simulink model "BMSController"  (R2026b)
undefined symbols (not defined in the file): BalNotActWait, BalOffWait, BalOnWait, BatteryLUT, contactorTime, currentFactor, CV_Gain, DiscIntNeverNeededParam, flgEnBalancing, HighTempLimit, I_cc, LowTempLimit, MaxCellVoltThrsld, MaxChrgCurrLim, MaxDchrgCurrLim, noCurrent, OverCellVoltageLimit, PlntBattChrgMax, PlntBattNumCellPar, PlntBattNumCellSer, PlntBattSocInit, PlntBattTempInitDegC, SnsrFltThld, TargetDeltaV, timeoutContactor, timeoutCurrent, UnderCellVoltageLimit, voltThreshold, vRatio
settings Model: Creator=The MathWorks, Inc.  LastModifiedBy=The MathWorks, Inc.

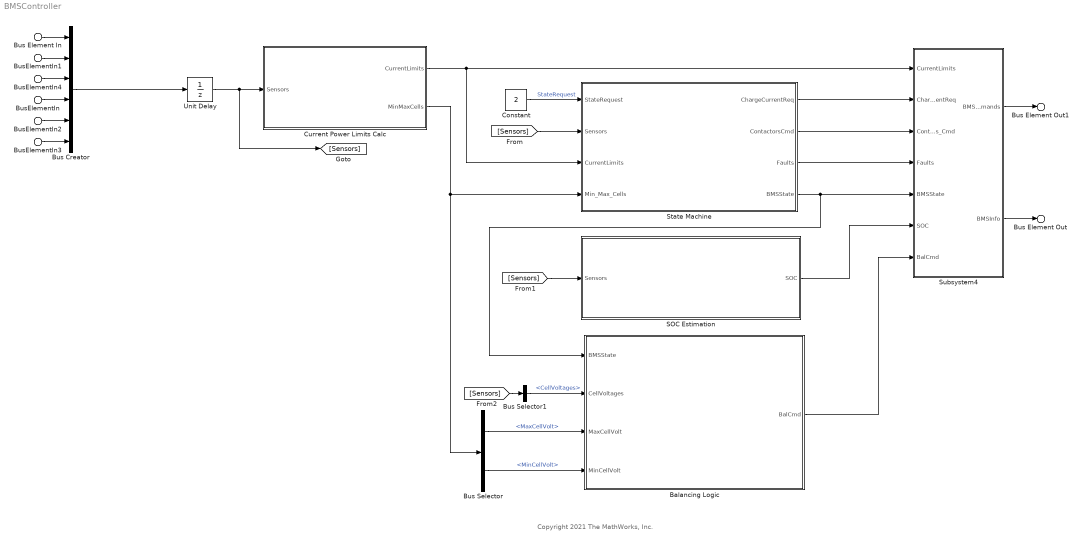
== system BMSController ==
  note: Copyright 2021 The MathWorks, Inc.
  Bus Element In : Inport  PortName=BMSSensors  Element=CellVoltages
  BusElementIn : Inport  PortName=BMSSensors  Element=CellTemperatures
  BusElementIn1 : Inport  PortName=BMSSensors  Element=PackVoltage
  BusElementIn2 : Inport  PortName=BMSSensors  Element=VoutChgr
  BusElementIn3 : Inport  PortName=BMSSensors  Element=VoutInvtr
  BusElementIn4 : Inport  PortName=BMSSensors  Element=PackCurrent
  Balancing Logic : Subsystem
  Bus Creator : BusCreator  Inputs=6
  Bus Selector : BusSelector  OutputSignals=MaxCellVolt,MinCellVolt
  Bus Selector1 : BusSelector  OutputSignals=CellVoltages
  Constant : Constant  Value=2  OutDataTypeStr=single  SampleTime=-1
  Current Power Limits Calc : Subsystem
  SOC Estimation : Subsystem
  State Machine : Subsystem
  Subsystem4 : Subsystem
  Unit Delay : UnitDelay  InitialCondition=struct('CellVoltages',3.6*ones(1, PlntBattNumCellSer),'PackVoltage',3.6*PlntBattNumCellSer,'PackCurrent',0,'CellTemperatures',PlntBattTempInitDegC*ones(1,PlntBattNumCellSer),'VoutChgr',0,'VoutInvtr',0)  SampleTime=-1
  Bus Element Out : Outport  PortName=BMSInfo
  Bus Element Out1 : Outport  Port=2  PortName=BMSCmd
  wires:
  State Machine/4(BMSState) -> Balancing Logic/1(BMSState), Subsystem4/5(BMSState)
  Constant/1 -> State Machine/1(StateRequest)  "StateRequest"
  Bus Selector1/1 -> Balancing Logic/2(CellVoltages)  "<CellVoltages>"
  SOC Estimation/1(SOC) -> Subsystem4/6(SOC)
  Balancing Logic/1(BalCmd) -> Subsystem4/7(BalCmd)
  Subsystem4/1(BMSCommands) -> Bus Element Out1/1
  Subsystem4/2(BMSInfo) -> Bus Element Out/1
  Current Power Limits Calc/1(CurrentLimits) -> State Machine/3(CurrentLimits), Subsystem4/1(CurrentLimits)
  State Machine/2(ContactorsCmd) -> Subsystem4/3(Contactors_Cmd)
  State Machine/1(ChargeCurrentReq) -> Subsystem4/2(ChargeCurrentReq)
  State Machine/3(Faults) -> Subsystem4/4(Faults)
  [Sensors] -> State Machine/2(Sensors)
  Current Power Limits Calc/2(MinMaxCells) -> State Machine/4(Min_Max_Cells), Bus Selector/1
  Bus Selector/1 -> Balancing Logic/3(MaxCellVolt)  "<MaxCellVolt>"
  Bus Selector/2 -> Balancing Logic/4(MinCellVolt)  "<MinCellVolt>"
  [Sensors] -> Bus Selector1/1
  Unit Delay/1 -> Current Power Limits Calc/1(Sensors), [Sensors]
  BusElementIn2/1 -> Bus Creator/5
  BusElementIn/1 -> Bus Creator/4
  Bus Element In/1 -> Bus Creator/1
  BusElementIn1/1 -> Bus Creator/2
  BusElementIn3/1 -> Bus Creator/6
  BusElementIn4/1 -> Bus Creator/3
  Bus Creator/1 -> Unit Delay/1
  [Sensors] -> SOC Estimation/1(Sensors)

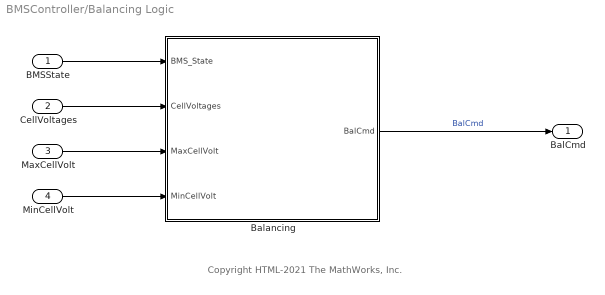
== system BMSController/Balancing Logic ==
  note: Copyright HTML-2021 The MathWorks, Inc.
  BMSState : Inport  OutDataTypeStr=single  PortDimensions=1  SampleTime=[5,0]
  CellVoltages : Inport  Port=2  OutDataTypeStr=single  PortDimensions=PlntBattNumCellSer  SampleTime=[5,0]
  MaxCellVolt : Inport  Port=3  OutDataTypeStr=single
  MinCellVolt : Inport  Port=4  OutDataTypeStr=single
  Balancing : Stateflow chart  TreatAsAtomicUnit=on  VariantControl=(default)
  BalCmd : Outport  OutDataTypeStr=boolean  PortDimensions=[1, PlntBattNumCellSer]  SampleTime=[5,0]  VectorParamsAs1DForOutWhenUnconnected=off
  wires:
  MinCellVolt/1 -> Balancing/4(MinCellVolt)
  MaxCellVolt/1 -> Balancing/3(MaxCellVolt)
  Balancing/1(BalCmd) -> BalCmd/1  "BalCmd"
  BMSState/1 -> Balancing/1(BMS_State)
  CellVoltages/1 -> Balancing/2(CellVoltages)

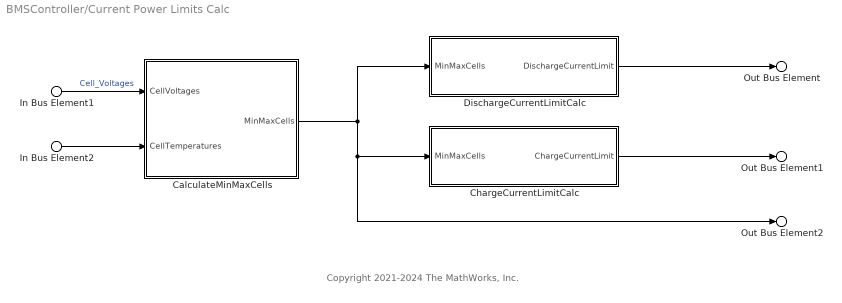
== system BMSController/Current Power Limits Calc ==
  note: Copyright 2021-2024 The MathWorks, Inc.
  In Bus Element1 : Inport  PortName=Sensors  Element=CellVoltages
  In Bus Element2 : Inport  PortName=Sensors  Element=CellTemperatures
  CalculateMinMaxCells : Subsystem
  ChargeCurrentLimitCalc : Subsystem
  DischargeCurrentLimitCalc : Subsystem
  Out Bus Element : Outport  PortName=CurrentLimits  Element=DischargeCurrentLimit
  Out Bus Element1 : Outport  PortName=CurrentLimits  Element=ChargeCurrentLimit
  Out Bus Element2 : Outport  Port=2  PortName=MinMaxCells
  wires:
  In Bus Element1/1 -> CalculateMinMaxCells/1(CellVoltages)  "Cell_Voltages"
  ChargeCurrentLimitCalc/1(ChargeCurrentLimit) -> Out Bus Element1/1
  In Bus Element2/1 -> CalculateMinMaxCells/2(CellTemperatures)
  CalculateMinMaxCells/1(MinMaxCells) -> Out Bus Element2/1, ChargeCurrentLimitCalc/1(MinMaxCells), DischargeCurrentLimitCalc/1(MinMaxCells)
  DischargeCurrentLimitCalc/1(DischargeCurrentLimit) -> Out Bus Element/1

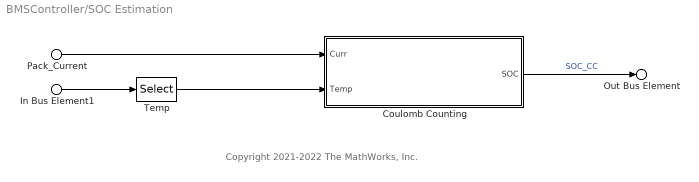
== system BMSController/SOC Estimation ==
  note: Copyright 2021-2022 The MathWorks, Inc.
  Pack_Current : Inport  PortName=Sensors  Element=PackCurrent
  In Bus Element1 : Inport  PortName=Sensors  Element=CellTemperatures
  Coulomb Counting : Subsystem  Variant=on  VariantControlMode=label  VariantControl=SocAlgo==1  LabelModeActiveChoice=Constant Capacity
  Temp : Selector  InputPortWidth=PlntBattNumCellSer  IndexOptions=Index vector (dialog)  Indices=1  OutputSizes=1  RuntimeRangeChecks=off
  Out Bus Element : Outport  PortName=SOC  Element=SOC_CC
  wires:
  Temp/1 -> Coulomb Counting/2(Temp)
  Pack_Current/1 -> Coulomb Counting/1(Curr)
  In Bus Element1/1 -> Temp/1
  Coulomb Counting/1(SOC) -> Out Bus Element/1  "SOC_CC"

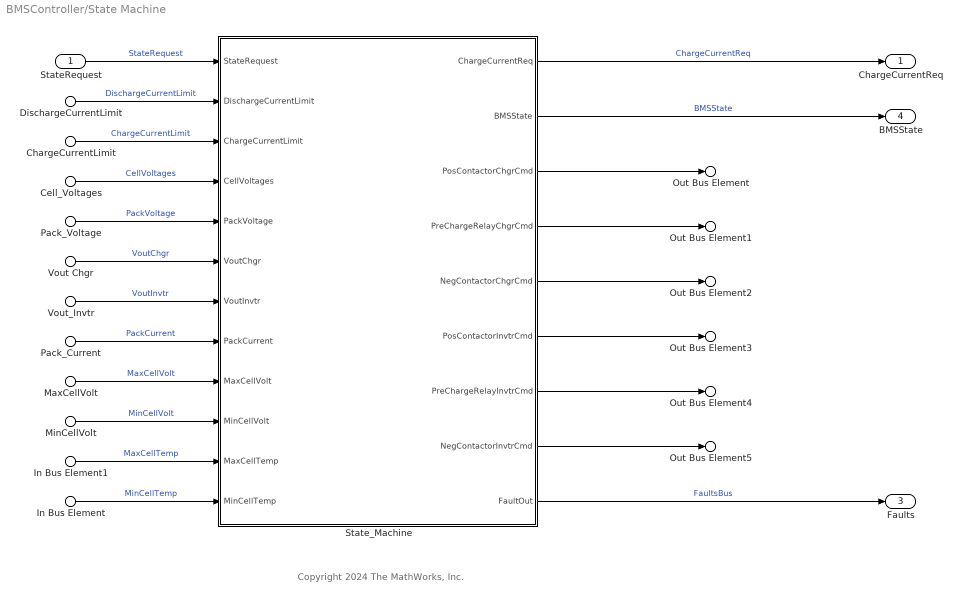
== system BMSController/State Machine ==
  note: Copyright 2024 The MathWorks, Inc.
  StateRequest : Inport  OutDataTypeStr=single  PortDimensions=1  SampleTime=[0.10000000000000001,0]
  Cell_Voltages : Inport  Port=2  PortName=Sensors  Element=CellVoltages
  Pack_Voltage : Inport  Port=2  PortName=Sensors  Element=PackVoltage
  Pack_Current : Inport  Port=2  PortName=Sensors  Element=PackCurrent
  Vout Chgr : Inport  Port=2  PortName=Sensors  Element=VoutChgr
  Vout_Invtr : Inport  Port=2  PortName=Sensors  Element=VoutInvtr
  DischargeCurrentLimit : Inport  Port=3  PortName=CurrentLimits  Element=DischargeCurrentLimit
  ChargeCurrentLimit : Inport  Port=3  PortName=CurrentLimits  Element=ChargeCurrentLimit
  MinCellVolt : Inport  Port=4  PortName=Min_Max_Cells  Element=MinCellVolt
  MaxCellVolt : Inport  Port=4  PortName=Min_Max_Cells  Element=MaxCellVolt
  In Bus Element : Inport  Port=4  PortName=Min_Max_Cells  Element=MinCellTemp
  In Bus Element1 : Inport  Port=4  PortName=Min_Max_Cells  Element=MaxCellTemp
  State_Machine : Stateflow chart  TreatAsAtomicUnit=on  VariantControl=(default)
  ChargeCurrentReq : Outport  OutMin=-100  OutMax=100  OutDataTypeStr=single  PortDimensions=1  SampleTime=[0.10000000000000001,0]  VectorParamsAs1DForOutWhenUnconnected=off
  Out Bus Element : Outport  Port=2  PortName=ContactorsCmd  Element=PosContactorChgrCmd
  Out Bus Element1 : Outport  Port=2  PortName=ContactorsCmd  Element=PreChargeRelayChgrCmd
  Out Bus Element2 : Outport  Port=2  PortName=ContactorsCmd  Element=NegContactorChgrCmd
  Out Bus Element3 : Outport  Port=2  PortName=ContactorsCmd  Element=PosContactorInvtrCmd
  Out Bus Element4 : Outport  Port=2  PortName=ContactorsCmd  Element=PreChargeRelayInvtrCmd
  Out Bus Element5 : Outport  Port=2  PortName=ContactorsCmd  Element=NegContactorInvtrCmd
  Faults : Outport  Port=3  OutDataTypeStr=boolean
  BMSState : Outport  Port=4  OutDataTypeStr=single  PortDimensions=1  SampleTime=[0.10000000000000001,0]  VectorParamsAs1DForOutWhenUnconnected=off
  wires:
  State_Machine/3(PosContactorChgrCmd) -> Out Bus Element/1
  In Bus Element/1 -> State_Machine/12(MinCellTemp)  "MinCellTemp"
  Pack_Voltage/1 -> State_Machine/5(PackVoltage)  "PackVoltage"
  State_Machine/4(PreChargeRelayChgrCmd) -> Out Bus Element1/1
  State_Machine/2(BMSState) -> BMSState/1  "BMSState"
  MaxCellVolt/1 -> State_Machine/9(MaxCellVolt)  "MaxCellVolt"
  MinCellVolt/1 -> State_Machine/10(MinCellVolt)  "MinCellVolt"
  Vout Chgr/1 -> State_Machine/6(VoutChgr)  "VoutChgr"
  ChargeCurrentLimit/1 -> State_Machine/3(ChargeCurrentLimit)  "ChargeCurrentLimit"
  In Bus Element1/1 -> State_Machine/11(MaxCellTemp)  "MaxCellTemp"
  Pack_Current/1 -> State_Machine/8(PackCurrent)  "PackCurrent"
  State_Machine/1(ChargeCurrentReq) -> ChargeCurrentReq/1  "ChargeCurrentReq"
  State_Machine/7(PreChargeRelayInvtrCmd) -> Out Bus Element4/1
  State_Machine/8(NegContactorInvtrCmd) -> Out Bus Element5/1
  State_Machine/6(PosContactorInvtrCmd) -> Out Bus Element3/1
  Cell_Voltages/1 -> State_Machine/4(CellVoltages)  "CellVoltages"
  State_Machine/5(NegContactorChgrCmd) -> Out Bus Element2/1
  StateRequest/1 -> State_Machine/1(StateRequest)  "StateRequest"
  State_Machine/9(FaultOut) -> Faults/1  "FaultsBus"
  DischargeCurrentLimit/1 -> State_Machine/2(DischargeCurrentLimit)  "DischargeCurrentLimit"
  Vout_Invtr/1 -> State_Machine/7(VoutInvtr)  "VoutInvtr"

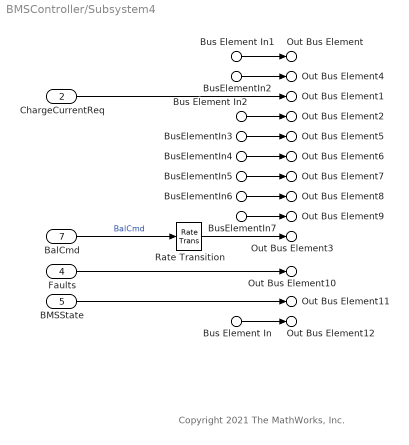
== system BMSController/Subsystem4 ==
  note: Copyright 2021 The MathWorks, Inc.
  Bus Element In1 : Inport  PortName=CurrentLimits  Element=DischargeCurrentLimit
  BusElementIn2 : Inport  PortName=CurrentLimits  Element=ChargeCurrentLimit
  ChargeCurrentReq : Inport  Port=2  OutDataTypeStr=single  PortDimensions=1  SampleTime=[0.10000000000000001,0]
  Bus Element In2 : Inport  Port=3  PortName=Contactors_Cmd  Element=PosContactorChgrCmd
  BusElementIn3 : Inport  Port=3  PortName=Contactors_Cmd  Element=PreChargeRelayChgrCmd
  BusElementIn4 : Inport  Port=3  PortName=Contactors_Cmd  Element=NegContactorChgrCmd
  BusElementIn5 : Inport  Port=3  PortName=Contactors_Cmd  Element=PosContactorInvtrCmd
  BusElementIn6 : Inport  Port=3  PortName=Contactors_Cmd  Element=PreChargeRelayInvtrCmd
  BusElementIn7 : Inport  Port=3  PortName=Contactors_Cmd  Element=NegContactorInvtrCmd
  Faults : Inport  Port=4  OutDataTypeStr=boolean
  BMSState : Inport  Port=5  OutDataTypeStr=single  PortDimensions=1  SampleTime=[0.10000000000000001,0]
  Bus Element In : Inport  Port=6  PortName=SOC  Element=SOC_CC
  BalCmd : Inport  Port=7  OutDataTypeStr=boolean  PortDimensions=[1 PlntBattNumCellSer]  SampleTime=[5,0]
  Rate Transition : RateTransition  Integrity=off  Deterministic=off
  Out Bus Element : Outport  PortName=BMSCommands  Element=CurrentLimitsBus.DischargeCurrentLimit
  Out Bus Element4 : Outport  PortName=BMSCommands  Element=CurrentLimitsBus.ChargeCurrentLimit
  Out Bus Element1 : Outport  PortName=BMSCommands  Element=ChargeCurrentReq
  Out Bus Element2 : Outport  PortName=BMSCommands  Element=ContactorsCmdBus.PosContactorChgrCmd
  Out Bus Element5 : Outport  PortName=BMSCommands  Element=ContactorsCmdBus.PreChargeRelayChgrCmd
  Out Bus Element6 : Outport  PortName=BMSCommands  Element=ContactorsCmdBus.NegContactorChgrCmd
  Out Bus Element7 : Outport  PortName=BMSCommands  Element=ContactorsCmdBus.PosContactorInvtrCmd
  Out Bus Element8 : Outport  PortName=BMSCommands  Element=ContactorsCmdBus.PreChargeRelayInvtrCmd
  Out Bus Element9 : Outport  PortName=BMSCommands  Element=ContactorsCmdBus.NegContactorInvtrCmd
  Out Bus Element3 : Outport  PortName=BMSCommands  Element=BalCmd
  Out Bus Element10 : Outport  Port=2  PortName=BMSInfo  Element=Faults
  Out Bus Element11 : Outport  Port=2  PortName=BMSInfo  Element=BMSState
  Out Bus Element12 : Outport  Port=2  PortName=BMSInfo  Element=SOC.SOC_CC
  wires:
  Bus Element In/1 -> Out Bus Element12/1
  Rate Transition/1 -> Out Bus Element3/1
  BusElementIn7/1 -> Out Bus Element9/1
  BusElementIn6/1 -> Out Bus Element8/1
  BusElementIn4/1 -> Out Bus Element6/1
  BusElementIn2/1 -> Out Bus Element4/1
  Faults/1 -> Out Bus Element10/1
  Bus Element In1/1 -> Out Bus Element/1
  BusElementIn3/1 -> Out Bus Element5/1
  BalCmd/1 -> Rate Transition/1  "BalCmd"
  ChargeCurrentReq/1 -> Out Bus Element1/1
  BMSState/1 -> Out Bus Element11/1
  Bus Element In2/1 -> Out Bus Element2/1
  BusElementIn5/1 -> Out Bus Element7/1

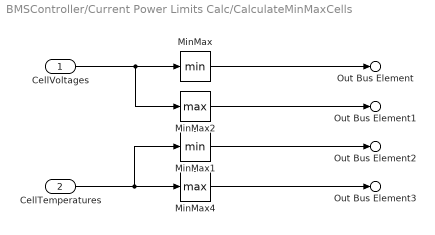
== system BMSController/Current Power Limits Calc/CalculateMinMaxCells ==
  CellVoltages : Inport
  CellTemperatures : Inport  Port=2
  MinMax : MinMax
  MinMax1 : MinMax
  MinMax2 : MinMax  Function=max
  MinMax4 : MinMax  Function=max
  Out Bus Element : Outport  PortName=MinMaxCells  Element=MinCellVolt
  Out Bus Element1 : Outport  PortName=MinMaxCells  Element=MaxCellVolt
  Out Bus Element2 : Outport  PortName=MinMaxCells  Element=MinCellTemp
  Out Bus Element3 : Outport  PortName=MinMaxCells  Element=MaxCellTemp
  wires:
  MinMax2/1 -> Out Bus Element1/1
  CellTemperatures/1 -> MinMax4/1, MinMax1/1
  MinMax/1 -> Out Bus Element/1
  CellVoltages/1 -> MinMax/1, MinMax2/1
  MinMax1/1 -> Out Bus Element2/1
  MinMax4/1 -> Out Bus Element3/1

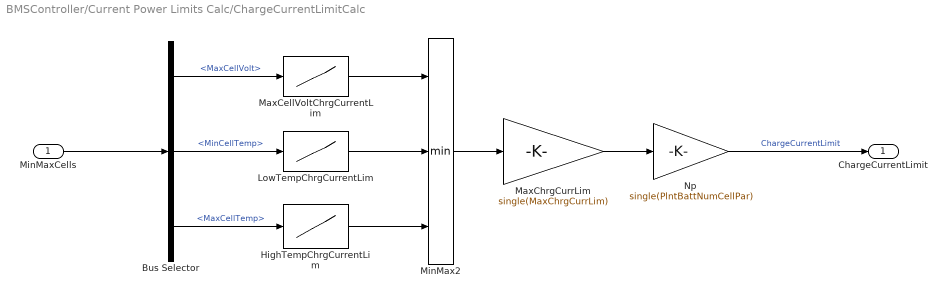
== system BMSController/Current Power Limits Calc/ChargeCurrentLimitCalc ==
  MinMaxCells : Inport
  Bus Selector : BusSelector  OutputSignals=MaxCellVolt,MinCellTemp,MaxCellTemp
  HighTempChrgCurrentLim : Lookup_n-D  NumberOfTableDimensions=1  BreakpointsForDimension1="single([40  45  50  55 60])"  Table=single([1.0 0.8 0.5 0.3 0])  ExtrapMethod=Clip  InternalRulePriority=Speed  RndMeth=Simplest
  LowTempChrgCurrentLim : Lookup_n-D  NumberOfTableDimensions=1  BreakpointsForDimension1=single([-15 -10 -5.0 0.0 5.0 10 15.0])  Table="single([0.1 0.2  0.3 0.3 0.5 1.0 1.0])"  ExtrapMethod=Clip  InternalRulePriority=Speed  RndMeth=Simplest
  MaxCellVoltChrgCurrentLim : Lookup_n-D  NumberOfTableDimensions=1  BreakpointsForDimension1=single([3.9 4.0 4.15 4.2])  Table="single([1.0 0.8 0.3  0.3])"  ExtrapMethod=Clip  InternalRulePriority=Speed  RndMeth=Simplest
  MaxChrgCurrLim : Gain  Gain=single(MaxChrgCurrLim)
  MinMax2 : MinMax  Inputs=3
  Np : Gain  Gain=single(PlntBattNumCellPar)
  ChargeCurrentLimit : Outport  VectorParamsAs1DForOutWhenUnconnected=off
  wires:
  MinMax2/1 -> MaxChrgCurrLim/1
  HighTempChrgCurrentLim/1 -> MinMax2/3
  LowTempChrgCurrentLim/1 -> MinMax2/2
  MaxChrgCurrLim/1 -> Np/1
  MinMaxCells/1 -> Bus Selector/1
  Bus Selector/2 -> LowTempChrgCurrentLim/1  "<MinCellTemp>"
  Bus Selector/3 -> HighTempChrgCurrentLim/1  "<MaxCellTemp>"
  MaxCellVoltChrgCurrentLim/1 -> MinMax2/1
  Bus Selector/1 -> MaxCellVoltChrgCurrentLim/1  "<MaxCellVolt>"
  Np/1 -> ChargeCurrentLimit/1  "ChargeCurrentLimit"

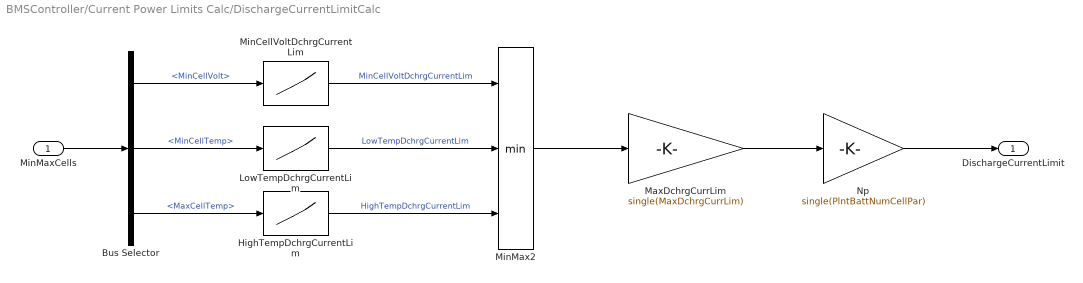
== system BMSController/Current Power Limits Calc/DischargeCurrentLimitCalc ==
  MinMaxCells : Inport
  Bus Selector : BusSelector  OutputSignals=MinCellVolt,MinCellTemp,MaxCellTemp
  HighTempDchrgCurrentLim : Lookup_n-D  NumberOfTableDimensions=1  BreakpointsForDimension1=single([40, 45, 50, 60])  Table=single([1, 0.5, 0.3, 0])  ExtrapMethod=Clip  InternalRulePriority=Speed  RndMeth=Simplest
  LowTempDchrgCurrentLim : Lookup_n-D  NumberOfTableDimensions=1  BreakpointsForDimension1="single([-10, -5,    0,   5, 10, 15, 20])"  Table="single([0,  0.2, 0.3, 0.5, 0.75, 1, 1])"  ExtrapMethod=Clip  InternalRulePriority=Speed  RndMeth=Simplest
  MaxDchrgCurrLim : Gain  Gain=single(MaxDchrgCurrLim)
  MinCellVoltDchrgCurrentLim : Lookup_n-D  NumberOfTableDimensions=1  LookupTableObject=MinCellVoltDchrgCurrentLimTable  BreakpointsForDimension1=single([2.5 2.75 3])  Table=single([0 0.5 1])  ExtrapMethod=Clip  InternalRulePriority=Speed  RndMeth=Simplest
  MinMax2 : MinMax  Inputs=3
  Np : Gain  Gain=single(PlntBattNumCellPar)
  DischargeCurrentLimit : Outport  VectorParamsAs1DForOutWhenUnconnected=off
  wires:
  MinMax2/1 -> MaxDchrgCurrLim/1
  MaxDchrgCurrLim/1 -> Np/1
  Bus Selector/3 -> HighTempDchrgCurrentLim/1  "<MaxCellTemp>"
  Bus Selector/2 -> LowTempDchrgCurrentLim/1  "<MinCellTemp>"
  HighTempDchrgCurrentLim/1 -> MinMax2/3  "HighTempDchrgCurrentLim"
  LowTempDchrgCurrentLim/1 -> MinMax2/2  "LowTempDchrgCurrentLim"
  Np/1 -> DischargeCurrentLimit/1
  MinMaxCells/1 -> Bus Selector/1
  MinCellVoltDchrgCurrentLim/1 -> MinMax2/1  "MinCellVoltDchrgCurrentLim"
  Bus Selector/1 -> MinCellVoltDchrgCurrentLim/1  "<MinCellVolt>"

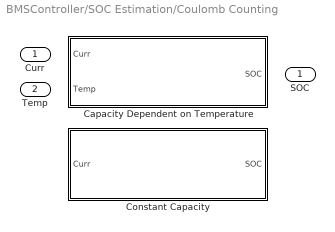
== system BMSController/SOC Estimation/Coulomb Counting ==
  Curr : Inport
  Temp : Inport  Port=2
  Capacity Dependent on Temperature : Subsystem  VariantControl=Capacity Dependent on Temperature
  Constant Capacity : Subsystem  VariantControl=Constant Capacity
  SOC : Outport

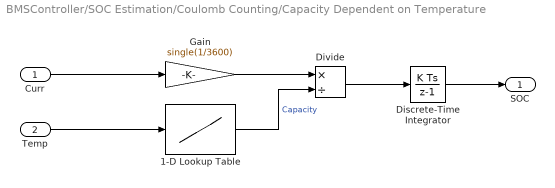
== system BMSController/SOC Estimation/Coulomb Counting/Capacity Dependent on Temperature ==
  Curr : Inport
  Temp : Inport  Port=2
  1-D Lookup Table : Lookup_n-D  NumberOfTableDimensions=1  BreakpointsForDimension1=single(BatteryLUT(1).Temperature_LUT)  Table=single(BatteryLUT(1).Capacity_LUT)*PlntBattNumCellPar  InternalRulePriority=Speed  RndMeth=Simplest
  Discrete-Time Integrator : DiscreteIntegrator  InitialCondition=single(PlntBattSocInit)  SampleTime=-1  LimitOutput=on  UpperSaturationLimit=1  LowerSaturationLimit=0  ICPrevOutput=DiscIntNeverNeededParam  ICPrevScaledInput=DiscIntNeverNeededParam
  Divide : Product  Inputs=*/
  Gain : Gain  Gain=single(1/3600)
  SOC : Outport  VectorParamsAs1DForOutWhenUnconnected=off
  wires:
  Discrete-Time Integrator/1 -> SOC/1
  Curr/1 -> Gain/1
  Gain/1 -> Divide/1
  Divide/1 -> Discrete-Time Integrator/1
  1-D Lookup Table/1 -> Divide/2  "Capacity"
  Temp/1 -> 1-D Lookup Table/1

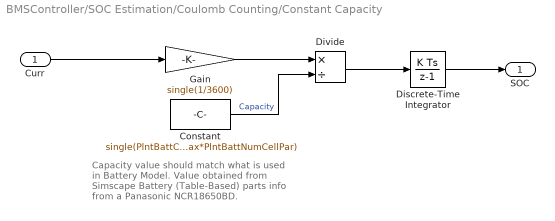
== system BMSController/SOC Estimation/Coulomb Counting/Constant Capacity ==
  note: Capacity value should match
      | what is used in Battery Model.
      | Value obtained from Simscape
      | Battery (Table-Based) parts info
      | from a Panasonic NCR18650BD.
  Curr : Inport  OutDataTypeStr=single
  Constant : Constant  Value=single(PlntBattChrgMax*PlntBattNumCellPar)  SampleTime=-1
  Discrete-Time Integrator : DiscreteIntegrator  InitialCondition=single(PlntBattSocInit)  SampleTime=-1  LimitOutput=on  UpperSaturationLimit=1  LowerSaturationLimit=0  ICPrevOutput=DiscIntNeverNeededParam  ICPrevScaledInput=DiscIntNeverNeededParam
  Divide : Product  Inputs=*/
  Gain : Gain  Gain=single(1/3600)
  SOC : Outport  VectorParamsAs1DForOutWhenUnconnected=off
  wires:
  Constant/1 -> Divide/2  "Capacity"
  Divide/1 -> Discrete-Time Integrator/1
  Gain/1 -> Divide/1
  Curr/1 -> Gain/1
  Discrete-Time Integrator/1 -> SOC/1

== stateflow chart BMSController/Balancing Logic/Balancing ==
  state BalancingOFF
    en:
    BalCmd(:,:) = false;
    en,du:
    DeltaCellVolt = MaxCellVolt - MinCellVolt;
  state BalancingON
    en, du:
    DeltaCellVolt = MaxCellVolt - MinCellVolt;
    state BalActive
      en, du:
      BalCmd = ((CellVoltages - MinCellVolt) > TargetDeltaV/2)';
      flgBalCompl = all(~BalCmd);
    state BalNotActive
    (default) -> BalActive
    BalNotActive -> BalActive [order 1] : [after(BalNotActWait,sec) && ...
        | DeltaCellVolt > TargetDeltaV]
    BalActive -> BalNotActive : [flgBalCompl]
  (default) -> BalancingOFF : {flgBalCompl = true;}
  BalancingOFF -> BalancingON : [flgEnBalancing && ...
      | BMS_State ~= 2 && ...
      | after(BalOffWait,sec) && ...
      | DeltaCellVolt > TargetDeltaV]
  BalancingON -> BalancingOFF : [BMS_State == 2]
      | %In Driving State
  BalNotActive -> BalancingOFF [order 2] : [after(BalOnWait,sec)]
  data: BMS_State input; CellVoltages input single; TargetDeltaV parameter; BalCmd output boolean size=[1, PlntBattNumCellSer] =boolean(zeros(1, PlntBattNumCellSer)); flgBalCompl local; MaxCellVolt input single; MinCellVolt input single; BalNotActWait parameter; BalOffWait parameter; BalOnWait parameter; flgEnBalancing parameter; DeltaCellVolt local single =single(0)

== stateflow chart BMSController/State Machine/State_Machine ==
  state Fault Monitoring [group]
    state MonitorCurrLim [parallel]
      settings: executionOrder=1
      state Wait
      state NoCurrLimFault
      state OverCurrentFault
        en:
        FaultPresent = true;
        FaultOut = true;
      (default) -> NoCurrLimFault : {FaultPresent = false;
          | FaultOut = false;}
      NoCurrLimFault -> Wait : [(PackCurrent < DischargeCurrentLimit) || ...
          | (PackCurrent > ChargeCurrentLimit)]
      Wait -> NoCurrLimFault [order 2] : [(PackCurrent >= DischargeCurrentLimit) && ...
          | (PackCurrent <= ChargeCurrentLimit)]
      Wait -> OverCurrentFault [order 1] : [after(timeoutCurrent,sec)]
    state MonitorCellVoltage [parallel]
      settings: executionOrder=2
      state OverVoltageFault
        en:
        FaultPresent = true;
        FaultOut = true;
      state NoCellVoltFault
        en,du:
        Delta = abs(PackVoltage - sum(CellVoltages));
      state SensorFaut
        en:
        FaultPresent = true;
        FaultOut = true;
      state UnderVoltageFault
        en:
        FaultPresent = true;
        FaultOut = true;
      (default) -> NoCellVoltFault : {FaultPresent = false;
          | FaultOut = false;
          | }
      NoCellVoltFault -> OverVoltageFault [order 1] : [MaxCellVolt >= ...
          | OverCellVoltageLimit]
      NoCellVoltFault -> SensorFaut [order 2] : [Delta >=...
          |  single(SnsrFltThld)]
      NoCellVoltFault -> UnderVoltageFault [order 3] : [MinCellVolt <=...
          |  UnderCellVoltageLimit]
    state MonitorCellTemp [parallel]
      settings: executionOrder=3
      state HighTemperatureFault
        en:
        FaultPresent = true;
        FaultOut = true;
      state NoCellTempFault
      state LowTemperatureFault
        en:
        FaultPresent = true;
        FaultOut = true;
      (default) -> NoCellTempFault : {FaultPresent = false;
          | FaultOut = false;}
      NoCellTempFault -> HighTemperatureFault [order 1] : [MaxCellTemp >= HighTempLimit]
      NoCellTempFault -> LowTemperatureFault [order 2] : [MinCellTemp <= LowTempLimit]
  state MainStateMachine [parallel]
    settings: executionOrder=1
    state Charging
      en:
      BMSState = 1;
      state Init_Mode
        en:
        ChargeModeReq = 0;
        ChargeCurrentReq = noCurrent;
      state CC_Mode
        en:
        ChargeModeReq = 1;
        du:
        ChargeCurrentReq = min(I_cc,ChargeCurrentLimit);
      state CV_Mode
        en:
        ChargeModeReq = 2;
        du:
        ChargeCurrentReq = ChargeCurrentReq - CV_Gain*(MaxCellVolt - MaxCellVoltThrsld);
        ChargeCurrentReq = min(ChargeCurrentReq, ChargeCurrentLimit);
      (default) -> Init_Mode
      CV_Mode -> Init_Mode : [StateRequest ~= 1 || ...
          | ChargeCurrentReq <= (I_cc/currentFactor)]
      CC_Mode -> Init_Mode [order 1] : [StateRequest ~= 1]
      Init_Mode -> CC_Mode : [StateRequest == 1 && ...
          | MaxCellVolt < voltThreshold]
      CC_Mode -> CV_Mode [order 2] : [MaxCellVolt>=...
          | MaxCellVoltThrsld]
    state Standby
      en:
      BMSState = ...
      0;
    state Driving
      en:
      BMSState = ...
      2;
    state Fault
      en,du:
      BMSState = 3;
    (default) -> Standby
    Standby -> (junction 577) [order 1] : [FaultPresent]
    Standby -> Charging [order 2] : [StateRequest ==1 ...
        | && ChrgCntctState == Contact.Close]
    (junction 577) -> (junction 580)
    Charging -> Standby [order 3] : [StateRequest ~=1 ...
        |  && ChrgCntctState == Contact.Init]
    Standby -> Driving [order 3] : [StateRequest == 2 && ...
        | InvtrCntctState == Contact.Close]
    Driving -> Standby [order 3] : [StateRequest ~= 2 && ...
        | InvtrCntctState == Contact.Init]
    Driving -> Charging [order 2] : [StateRequest == 1 && ...
        | ChrgCntctState == Contact.Close]
    Charging -> Driving [order 2] : [StateRequest == 2 && ...
        | InvtrCntctState == Contact.Close]
    Driving -> Fault [order 1] : [FaultPresent]
    Charging -> Fault [order 1] : [FaultPresent]{ChargeCurrentReq = single(0);}
    (junction 580) -> Fault
  state ChargerContactorState [parallel]
    settings: executionOrder=2
    state OpenChgrContactors
      state ClosePreChrgRly
        PreChargeRelayChgrCmd = true;
      state OpenPosCntct
        PosContactorChgrCmd = false;
      state OpenPreChrgRly
        PreChargeRelayChgrCmd = false;
      state OpenNegCntct
        NegContactorChgrCmd = false;
        ChrgCntctState = Contact.Open;
        PreChrgFault = false;
        FaultOut = false;
      (default) -> ChargerContactorState.OpenChgrContactors.ClosePreChrgRly : {ChrgCntctState = Contact.Init;}
      ChargerContactorState.OpenChgrContactors.ClosePreChrgRly -> ChargerContactorState.OpenChgrContactors.OpenPosCntct : after(contactorTime,msec) % Check for low current
      ChargerContactorState.OpenChgrContactors.OpenPosCntct -> ChargerContactorState.OpenChgrContactors.OpenPreChrgRly : after(contactorTime,msec)
      ChargerContactorState.OpenChgrContactors.OpenPreChrgRly -> ChargerContactorState.OpenChgrContactors.OpenNegCntct : after(contactorTime,msec)
    state CloseChgrContactors
      state CloseNegCntct
        NegContactorChgrCmd = true;
      state ClosePreChrgRly
        PreChargeRelayChgrCmd = true;
      state ClosePosCntct
        PosContactorChgrCmd = true;
      state OpenPreChrgRly
        PreChargeRelayChgrCmd = false;
        ChrgCntctState = Contact.Close;
      state PreChrgFlt
        PreChrgFault = true;
        FaultOut = true;
      (default) -> ChargerContactorState.CloseChgrContactors.CloseNegCntct : {ChrgCntctState = Contact.Init;}
      ChargerContactorState.CloseChgrContactors.CloseNegCntct -> ChargerContactorState.CloseChgrContactors.ClosePreChrgRly : after(contactorTime,msec)
      ChargerContactorState.CloseChgrContactors.ClosePreChrgRly -> (junction 564) [order 2]
      (junction 564) -> (junction 566) : after(timeoutContactor,sec)
          | % Check timeout
      ChargerContactorState.CloseChgrContactors.ClosePreChrgRly -> ChargerContactorState.CloseChgrContactors.ClosePosCntct [order 1] : [VoutChgr/PackVoltage >=vRatio]
      ChargerContactorState.CloseChgrContactors.ClosePosCntct -> ChargerContactorState.CloseChgrContactors.OpenPreChrgRly : after(contactorTime,msec)
      (junction 566) -> ChargerContactorState.CloseChgrContactors.PreChrgFlt
    (default) -> OpenChgrContactors : {ChrgCntctState = Contact.Init;
        | PreChrgFault = false;
        | FaultOut = false;}
    CloseChgrContactors -> OpenChgrContactors : [StateRequest ~= 1 || ...
        | FaultPresent]
    OpenChgrContactors -> CloseChgrContactors : [StateRequest == 1 && ...
        | InvtrCntctState == Contact.Open && ...
        | ~FaultPresent]
  state InverterContactorState [parallel]
    settings: executionOrder=3
    state CloseInvtrContactors
      state CloseNegCntct
        NegContactorInvtrCmd = true;
      state ClosePreChrgRly
        PreChargeRelayInvtrCmd = true;
      state ClosePosCntct
        PosContactorInvtrCmd = true;
      state OpenPreChrgRly
        PreChargeRelayInvtrCmd = false;
        InvtrCntctState = Contact.Close;
      state PreChrgFlt
        PreChrgFault = true;
        FaultOut = true;
      (default) -> InverterContactorState.CloseInvtrContactors.CloseNegCntct : {InvtrCntctState = Contact.Init;}
      InverterContactorState.CloseInvtrContactors.CloseNegCntct -> InverterContactorState.CloseInvtrContactors.ClosePreChrgRly : after(contactorTime,msec)
      InverterContactorState.CloseInvtrContactors.ClosePreChrgRly -> (junction 569) [order 2]
      (junction 569) -> (junction 570) : after(timeoutContactor,sec)
          | % Check timeout
      InverterContactorState.CloseInvtrContactors.ClosePreChrgRly -> InverterContactorState.CloseInvtrContactors.ClosePosCntct [order 1] : [VoutInvtr/PackVoltage >=vRatio]
      InverterContactorState.CloseInvtrContactors.ClosePosCntct -> InverterContactorState.CloseInvtrContactors.OpenPreChrgRly : after(contactorTime,msec)
      (junction 570) -> InverterContactorState.CloseInvtrContactors.PreChrgFlt
    state OpenInvtrContactors
      state ClosePreChrgRly
        PreChargeRelayInvtrCmd = true;
      state OpenPosCntct
        PosContactorInvtrCmd = false;
      state OpenPreChrgRly
        PreChargeRelayInvtrCmd = false;
      state OpenNegCntct
        NegContactorInvtrCmd = false;
        InvtrCntctState = Contact.Open;
        PreChrgFault = false;
        FaultOut = false;
      (default) -> InverterContactorState.OpenInvtrContactors.ClosePreChrgRly : {InvtrCntctState = Contact.Init;}
      InverterContactorState.OpenInvtrContactors.ClosePreChrgRly -> InverterContactorState.OpenInvtrContactors.OpenPosCntct : after(contactorTime,msec) % Check for low current
      InverterContactorState.OpenInvtrContactors.OpenPosCntct -> InverterContactorState.OpenInvtrContactors.OpenPreChrgRly : after(contactorTime,msec)
      InverterContactorState.OpenInvtrContactors.OpenPreChrgRly -> InverterContactorState.OpenInvtrContactors.OpenNegCntct : after(contactorTime,msec)
    (default) -> OpenInvtrContactors : {InvtrCntctState =Contact.Init;
        | PreChrgFault = false;
        | FaultOut = false;}
    CloseInvtrContactors -> OpenInvtrContactors : [StateRequest ~= 2 || ...
        | FaultPresent]
    OpenInvtrContactors -> CloseInvtrContactors : [StateRequest == 2 && ...
        | ChrgCntctState == Contact.Open && ...
        | ~FaultPresent]
  data: StateRequest input; DischargeCurrentLimit input single; ChargeCurrentLimit input single; CellVoltages input single; PackVoltage input single; VoutChgr input single; VoutInvtr input single; PackCurrent input single; ChargeCurrentReq output single; I_cc parameter; MaxCellVolt input single; BMSState output single =single(0); PosContactorChgrCmd output boolean; PreChargeRelayChgrCmd output; NegContactorChgrCmd output; PosContactorInvtrCmd output; PreChargeRelayInvtrCmd output; NegContactorInvtrCmd output; ChrgCntctState local Enum: Contact; InvtrCntctState local Enum: Contact; PreChrgFault local; MaxCellVoltThrsld parameter; FaultPresent local; MinCellVolt input single; OverCellVoltageLimit parameter; UnderCellVoltageLimit parameter; Delta local; HighTempLimit parameter; LowTempLimit parameter; SnsrFltThld parameter; CV_Gain parameter; ChargeModeReq local =0; MonitorCurrLimMode local Enum: MonitorCurrLimModeType; MonitorCellVoltageMode local Enum: MonitorCellVoltageModeType; MonitorCellTempMode local Enum: MonitorCellTempModeType; FaultOut output boolean; contactorTime parameter uint16; timeoutContactor parameter uint8; timeoutCurrent parameter uint8; vRatio parameter single; voltThreshold parameter single; currentFactor parameter single; noCurrent parameter single; MaxCellTemp input; MinCellTemp input
